simulink model "momentumBasedFlying"  (Simulink 10.2)
settings: Solver=FixedStepAuto  StartTime=0.0  StopTime=Config.simulationTime  FixedStep=Config.tStep  RelTol=1e-3
InitFcn:
  | cd(fileparts(which(bdroot)));
  | initMomentumBasedFlying;
StopFcn:
  | cd(fileparts(which(bdroot)));
  | stopMomentumBasedFlying;
undefined symbols (not defined in the file or in its folder): biasVectorConstraint_feet, Config, confVisualizer, ConstraintMatrix_feet, DiscIntNeverNeededParam, jets_config
libraries: WBToolboxLibrary x85
(part 4 of 4)

== matlab function iRonCub/Forward Dynamics/old_simulator_subsystem/State Integration/Homogeneous_matrix  ==
  data: p input double; H output double; R input double
function H = Rp2Hom(p, R)
    H = Rp2Hom(R, p);
end

== matlab function FLYING CONTROLLER (CORE) V2.5/Flying Controller v2.5/Momentum Control for Flying/Feedback linearization/MATLAB Function ==
  data: jets input double; jets_dot input double; jets_dot_des input double; throttle output double size=[4,1]; Config parameter double; error output double; integral_err input double
function [throttle, error]  = fl_jet_control(jets, jets_dot, jets_dot_des, Config, integral_err)

[throttle, error]  = fl_jet_control(jets, jets_dot, jets_dot_des, Config, integral_err);
end

== matlab function FLYING CONTROLLER (CORE) V2.5/Flying Controller v2.5/Momentum Control for Flying/extendedKalmanFilter4jets/EKF_jet2/EKF  ==
  data: x input double; input input double; measurement input double; xDot output double; P input double; Config parameter double; Pdot output double
function [xDot, Pdot] = extendedKalmanFilterFNC(x, input, measurement, P, Config)

[xDot, Pdot] = extKalmanFilter(x, input, Config.jetC_P100, P, measurement, Config);

== matlab function FLYING CONTROLLER (CORE) V2.5/Flying Controller v2.5/Momentum Control for Flying/extendedKalmanFilter4jets/EKF_jet2/splitVector ==
  data: x input double; x1 output double; x2 output double
function [x1, x2] = fcn(x)
x1 = x(1);
x2 = x(2);

== matlab function FLYING CONTROLLER (CORE) V2.5/Flying Controller v2.5/Momentum Control for Flying/extendedKalmanFilter4jets/EKF_jet3/EKF  ==
  data: x input double; input input double; measurement input double; xDot output double; P input double; Config parameter double; Pdot output double
function [xDot, Pdot] = extendedKalmanFilterFNC(x, input, measurement, P, Config)

[xDot, Pdot] = extKalmanFilter(x, input, Config.jetC_P220, P, measurement, Config);

== matlab function FLYING CONTROLLER (CORE) V2.5/Flying Controller v2.5/Momentum Control for Flying/extendedKalmanFilter4jets/EKF_jet3/splitVector ==
  data: x input double; x1 output double; x2 output double
function [x1, x2] = fcn(x)
x1 = x(1);
x2 = x(2);

== matlab function FLYING CONTROLLER (CORE) V2.5/Flying Controller v2.5/Momentum Control for Flying/extendedKalmanFilter4jets/EKF_jet4/EKF  ==
  data: x input double; input input double; measurement input double; xDot output double; P input double; Config parameter double; Pdot output double
function [xDot, Pdot] = extendedKalmanFilterFNC(x, input, measurement, P, Config)

[xDot, Pdot] = extKalmanFilter(x, input, Config.jetC_P220, P, measurement, Config);

== matlab function FLYING CONTROLLER (CORE) V2.5/Flying Controller v2.5/Momentum Control for Flying/extendedKalmanFilter4jets/EKF_jet4/splitVector ==
  data: x input double; x1 output double; x2 output double
function [x1, x2] = fcn(x)
x1 = x(1);
x2 = x(2);
